simulink model "full4bit"  (R2025b)
settings: Solver=VariableStepAuto  StartTime=0.0  StopTime=10.0  RelTol=1e-3
settings Model: Creator=cyber  LastModifiedBy=cyber

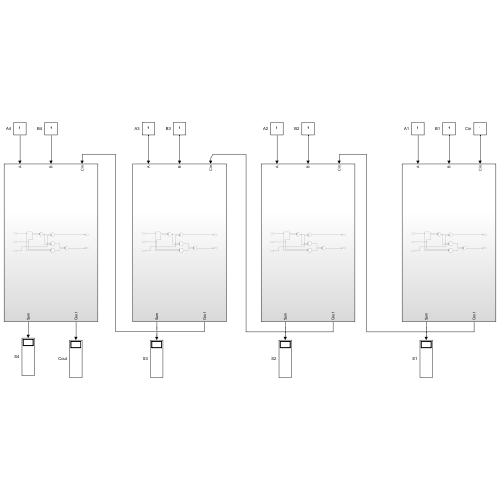
[thumbnail: Simulink's stored preview of the top-level diagram]
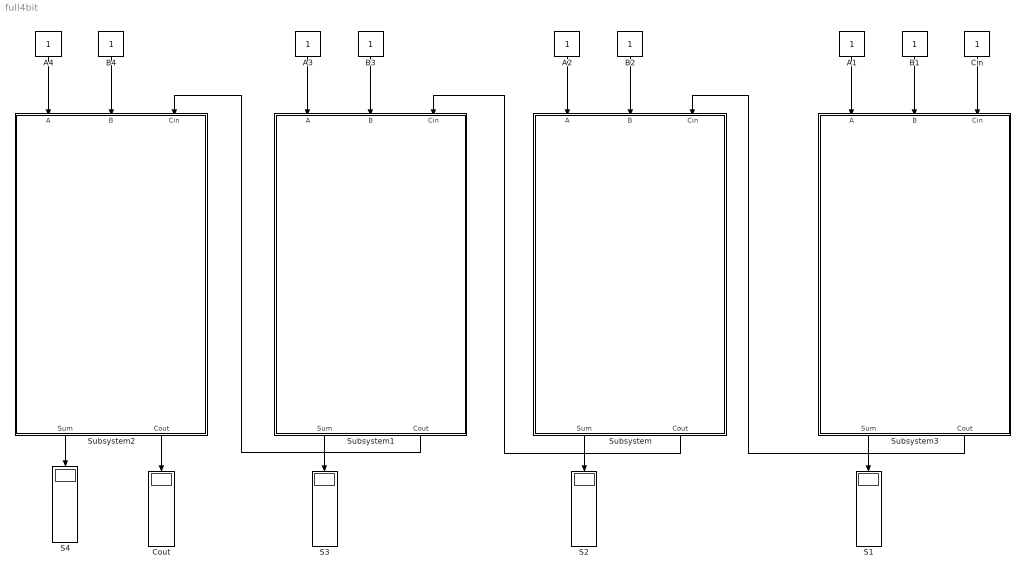
== system full4bit ==
  A{1..4} (4 alike) : Constant
  B{1..4} (4 alike) : Constant
  Cin : Constant
  Cout : Display
  S{1..4} (4 alike) : Display
  Subsystem : Subsystem
  Subsystem1 : Subsystem
  Subsystem2 : Subsystem
  Subsystem3 : Subsystem
  wires:
  Subsystem3/2(Cout) -> Subsystem/3(Cin)
  Subsystem/2(Cout) -> Subsystem1/3(Cin)
  Subsystem1/2(Cout) -> Subsystem2/3(Cin)
  A4/1 -> Subsystem2/1(A)
  B4/1 -> Subsystem2/2(B)
  A3/1 -> Subsystem1/1(A)
  B3/1 -> Subsystem1/2(B)
  A2/1 -> Subsystem/1(A)
  B2/1 -> Subsystem/2(B)
  A1/1 -> Subsystem3/1(A)
  B1/1 -> Subsystem3/2(B)
  Cin/1 -> Subsystem3/3(Cin)
  Subsystem2/1(Sum) -> S4/1
  Subsystem2/2(Cout) -> Cout/1
  Subsystem1/1(Sum) -> S3/1
  Subsystem/1(Sum) -> S2/1
  Subsystem3/1(Sum) -> S1/1

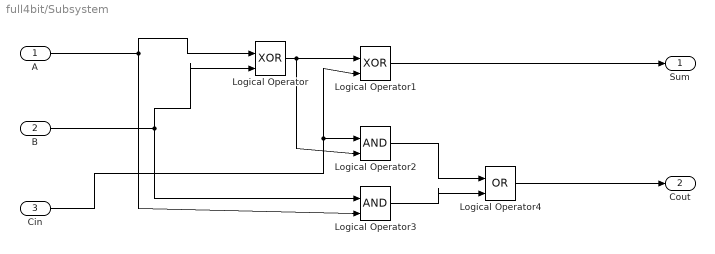
== system full4bit/Subsystem ==
  A : Inport
  B : Inport  Port=2
  Cin : Inport  Port=3
  Logical Operator : Logic  Operator=XOR  IconShape=distinctive  AllPortsSameDT=off  OutDataTypeStr=boolean
  Logical Operator1 : Logic  Operator=XOR  IconShape=distinctive  AllPortsSameDT=off  OutDataTypeStr=boolean
  Logical Operator2 : Logic  IconShape=distinctive  AllPortsSameDT=off  OutDataTypeStr=boolean
  Logical Operator3 : Logic  IconShape=distinctive  AllPortsSameDT=off  OutDataTypeStr=boolean
  Logical Operator4 : Logic  Operator=OR  IconShape=distinctive  AllPortsSameDT=off  OutDataTypeStr=boolean
  Sum : Outport
  Cout : Outport  Port=2
  wires:
  Logical Operator3/1 -> Logical Operator4/2
  B/1 -> Logical Operator/2, Logical Operator3/1
  Logical Operator/1 -> Logical Operator2/2, Logical Operator1/1
  Logical Operator1/1 -> Sum/1
  Logical Operator2/1 -> Logical Operator4/1
  Cin/1 -> Logical Operator2/1, Logical Operator1/2
  A/1 -> Logical Operator/1, Logical Operator3/2
  Logical Operator4/1 -> Cout/1

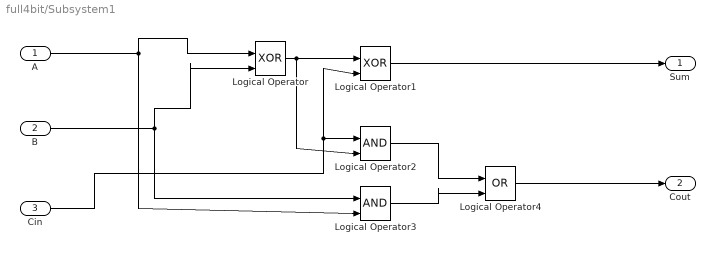
== system full4bit/Subsystem1 ==
  A : Inport
  B : Inport  Port=2
  Cin : Inport  Port=3
  Logical Operator : Logic  Operator=XOR  IconShape=distinctive  AllPortsSameDT=off  OutDataTypeStr=boolean
  Logical Operator1 : Logic  Operator=XOR  IconShape=distinctive  AllPortsSameDT=off  OutDataTypeStr=boolean
  Logical Operator2 : Logic  IconShape=distinctive  AllPortsSameDT=off  OutDataTypeStr=boolean
  Logical Operator3 : Logic  IconShape=distinctive  AllPortsSameDT=off  OutDataTypeStr=boolean
  Logical Operator4 : Logic  Operator=OR  IconShape=distinctive  AllPortsSameDT=off  OutDataTypeStr=boolean
  Sum : Outport
  Cout : Outport  Port=2
  wires:
  Logical Operator3/1 -> Logical Operator4/2
  B/1 -> Logical Operator/2, Logical Operator3/1
  Logical Operator/1 -> Logical Operator2/2, Logical Operator1/1
  Logical Operator1/1 -> Sum/1
  Logical Operator2/1 -> Logical Operator4/1
  Cin/1 -> Logical Operator2/1, Logical Operator1/2
  A/1 -> Logical Operator/1, Logical Operator3/2
  Logical Operator4/1 -> Cout/1

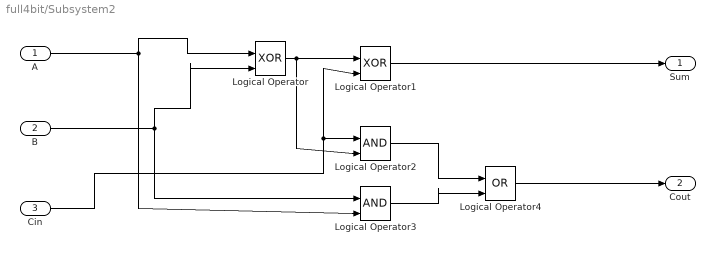
== system full4bit/Subsystem2 ==
  A : Inport
  B : Inport  Port=2
  Cin : Inport  Port=3
  Logical Operator : Logic  Operator=XOR  IconShape=distinctive  AllPortsSameDT=off  OutDataTypeStr=boolean
  Logical Operator1 : Logic  Operator=XOR  IconShape=distinctive  AllPortsSameDT=off  OutDataTypeStr=boolean
  Logical Operator2 : Logic  IconShape=distinctive  AllPortsSameDT=off  OutDataTypeStr=boolean
  Logical Operator3 : Logic  IconShape=distinctive  AllPortsSameDT=off  OutDataTypeStr=boolean
  Logical Operator4 : Logic  Operator=OR  IconShape=distinctive  AllPortsSameDT=off  OutDataTypeStr=boolean
  Sum : Outport
  Cout : Outport  Port=2
  wires:
  Logical Operator3/1 -> Logical Operator4/2
  B/1 -> Logical Operator/2, Logical Operator3/1
  Logical Operator/1 -> Logical Operator2/2, Logical Operator1/1
  Logical Operator1/1 -> Sum/1
  Logical Operator2/1 -> Logical Operator4/1
  Cin/1 -> Logical Operator2/1, Logical Operator1/2
  A/1 -> Logical Operator/1, Logical Operator3/2
  Logical Operator4/1 -> Cout/1

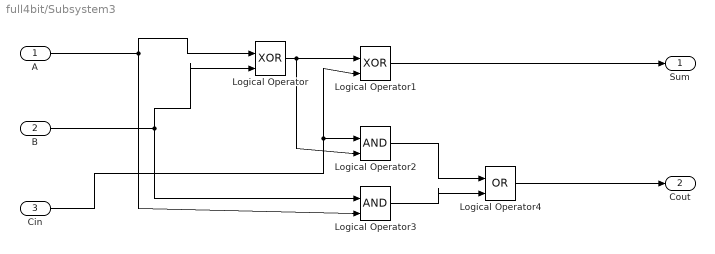
== system full4bit/Subsystem3 ==
  A : Inport
  B : Inport  Port=2
  Cin : Inport  Port=3
  Logical Operator : Logic  Operator=XOR  IconShape=distinctive  AllPortsSameDT=off  OutDataTypeStr=boolean
  Logical Operator1 : Logic  Operator=XOR  IconShape=distinctive  AllPortsSameDT=off  OutDataTypeStr=boolean
  Logical Operator2 : Logic  IconShape=distinctive  AllPortsSameDT=off  OutDataTypeStr=boolean
  Logical Operator3 : Logic  IconShape=distinctive  AllPortsSameDT=off  OutDataTypeStr=boolean
  Logical Operator4 : Logic  Operator=OR  IconShape=distinctive  AllPortsSameDT=off  OutDataTypeStr=boolean
  Sum : Outport
  Cout : Outport  Port=2
  wires:
  Logical Operator3/1 -> Logical Operator4/2
  B/1 -> Logical Operator/2, Logical Operator3/1
  Logical Operator/1 -> Logical Operator2/2, Logical Operator1/1
  Logical Operator1/1 -> Sum/1
  Logical Operator2/1 -> Logical Operator4/1
  Cin/1 -> Logical Operator2/1, Logical Operator1/2
  A/1 -> Logical Operator/1, Logical Operator3/2
  Logical Operator4/1 -> Cout/1
